simulink model "dynamic_model_soft_robot"  (R2018a)
settings: Solver=ode4  StartTime=0.0  StopTime=t_span  FixedStep=dt  RelTol=1e-3
values from neighbouring files (symbols this model uses):
  alpha0 = 0    [data_simulate_srm_dynamic_model.m]
  c1 = 0.12    [data_simulate_srm_dynamic_model.m]
  c2 = 5.93e-7    (= 5.93e-07)    [data_simulate_srm_dynamic_model.m]
  c3 = 5.93e-7    (= 5.93e-07)    [data_simulate_srm_dynamic_model.m]
  d0 = 0.0644    [data_simulate_srm_dynamic_model.m]
  dq_0 = [0; 0; 500]    [data_simulate_srm_dynamic_model.m]
  dt = 1.00e-03    (= 0.001)    [data_simulate_srm_dynamic_model.m]    (also in simulateSoftRobot.m)
  g = 9.81    [data_simulate_srm_dynamic_model.m]    (also in simulateSoftRobot.m)
  m = 0.0494    [data_simulate_srm_dynamic_model.m]    (also in simulateSoftRobot.m)
  noise_ddq = 0*[1e-4, 1e-4, 1e-4]    [data_simulate_srm_dynamic_model.m]
  noise_dq = 0*[1e-4, 1e-4, 1e-4]    [data_simulate_srm_dynamic_model.m]
  noise_q = 0*[1e-6, 1e-1, 1e-1]    [data_simulate_srm_dynamic_model.m]
  p_true = [b1; b2; b3; b4; b5; b6]    [data_simulate_srm_dynamic_model.m]
  q_0 = [d0; 10; .1]    [data_simulate_srm_dynamic_model.m]
  r = 0.0235    [data_simulate_srm_dynamic_model.m]    (also in simulateSoftRobot.m = 0.02)
libraries: dspinverses x1
(part 1 of 3)
settings Model: Creator=s118759  LastModifiedBy=s118759
settings CodeAppCC: StateflowObjectComments=on

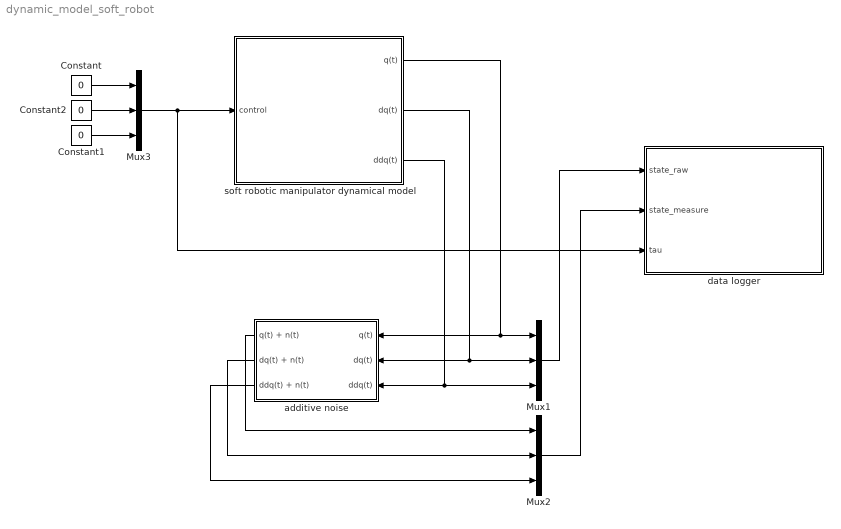
== system dynamic_model_soft_robot ==
  Constant : Constant  Value=0
  Constant1 : Constant  Value=0
  Constant2 : Constant  Value=0
  Mux1 : Mux  Inputs=3
  Mux2 : Mux  Inputs=3
  Mux3 : Mux  Inputs=3
  "additive noise " : Subsystem
  data logger : Subsystem
  soft robotic manipulator dynamical model : Subsystem
  wires:
  soft robotic manipulator dynamical model/1(q(t)) -> "additive noise "/1(q(t)), Mux1/1
  soft robotic manipulator dynamical model/2("dq(t) ") -> Mux1/2, "additive noise "/2(dq(t))
  soft robotic manipulator dynamical model/3("ddq(t) ") -> "additive noise "/3(ddq(t)), Mux1/3
  Mux1/1 -> data logger/1("state_raw ")
  "additive noise "/1(q(t) + n(t)) -> Mux2/1
  "additive noise "/2(dq(t) + n(t)) -> Mux2/2
  "additive noise "/3(ddq(t) + n(t)) -> Mux2/3
  Mux2/1 -> data logger/2(state_measure)
  Mux3/1 -> data logger/3(tau), soft robotic manipulator dynamical model/1("control ")
  Constant/1 -> Mux3/1
  Constant1/1 -> Mux3/3
  Constant2/1 -> Mux3/2

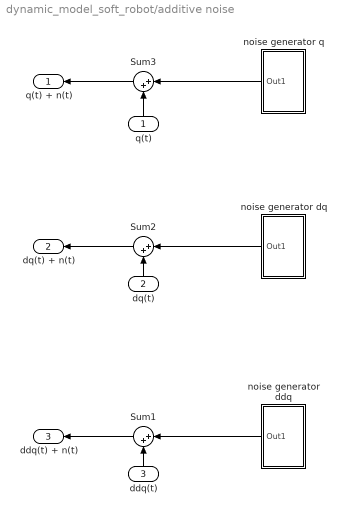
== system dynamic_model_soft_robot/additive noise  ==
  q(t) : Inport
  dq(t) : Inport  Port=2
  ddq(t) : Inport  Port=3
  Sum1 : Sum  Inputs=|++
  Sum2 : Sum  Inputs=|++
  Sum3 : Sum  Inputs=|++
  noise generator ddq : Subsystem
  noise generator dq : Subsystem
  noise generator q : Subsystem
  q(t) + n(t) : Outport
  dq(t) + n(t) : Outport  Port=2
  ddq(t) + n(t) : Outport  Port=3
  wires:
  Sum2/1 -> dq(t) + n(t)/1
  q(t)/1 -> Sum3/2
  Sum3/1 -> q(t) + n(t)/1
  dq(t)/1 -> Sum2/2
  Sum1/1 -> ddq(t) + n(t)/1
  ddq(t)/1 -> Sum1/2
  noise generator q/1(Out1) -> Sum3/1
  noise generator dq/1(Out1) -> Sum2/1
  noise generator ddq/1(Out1) -> Sum1/1

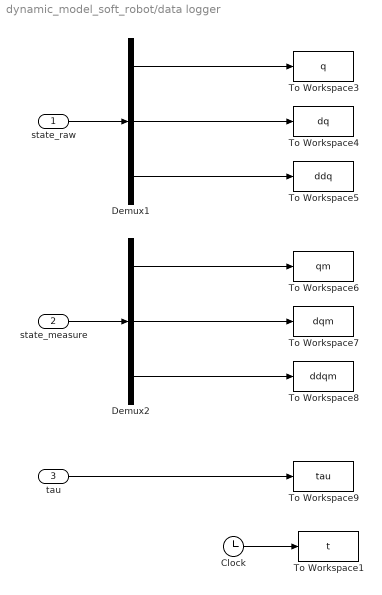
== system dynamic_model_soft_robot/data logger ==
  "state_raw " : Inport
  state_measure : Inport  Port=2
  tau : Inport  Port=3
  Clock : Clock
  Demux1 : Demux  Outputs=3
  Demux2 : Demux  Outputs=3
  To Workspace1 : ToWorkspace  VariableName=t  SampleTime=-1
      settings: Save2DSignal=2-D array (concatenate along first dimension)
  To Workspace3 : ToWorkspace  VariableName=q  SampleTime=-1
      settings: Save2DSignal=2-D array (concatenate along first dimension)
  To Workspace4 : ToWorkspace  VariableName=dq  SampleTime=-1
      settings: Save2DSignal=2-D array (concatenate along first dimension)
  To Workspace5 : ToWorkspace  VariableName=ddq  SampleTime=-1
      settings: Save2DSignal=2-D array (concatenate along first dimension)
  To Workspace6 : ToWorkspace  VariableName=qm  SampleTime=-1
      settings: Save2DSignal=2-D array (concatenate along first dimension)
  To Workspace7 : ToWorkspace  VariableName=dqm  SampleTime=-1
      settings: Save2DSignal=2-D array (concatenate along first dimension)
  To Workspace8 : ToWorkspace  VariableName=ddqm  SampleTime=-1
      settings: Save2DSignal=2-D array (concatenate along first dimension)
  To Workspace9 : ToWorkspace  VariableName=tau  SampleTime=-1
      settings: Save2DSignal=2-D array (concatenate along first dimension)
  wires:
  "state_raw "/1 -> Demux1/1
  Demux1/1 -> To Workspace3/1
  Demux1/2 -> To Workspace4/1
  Demux1/3 -> To Workspace5/1
  state_measure/1 -> Demux2/1
  Demux2/1 -> To Workspace6/1
  Demux2/2 -> To Workspace7/1
  Demux2/3 -> To Workspace8/1
  tau/1 -> To Workspace9/1
  Clock/1 -> To Workspace1/1

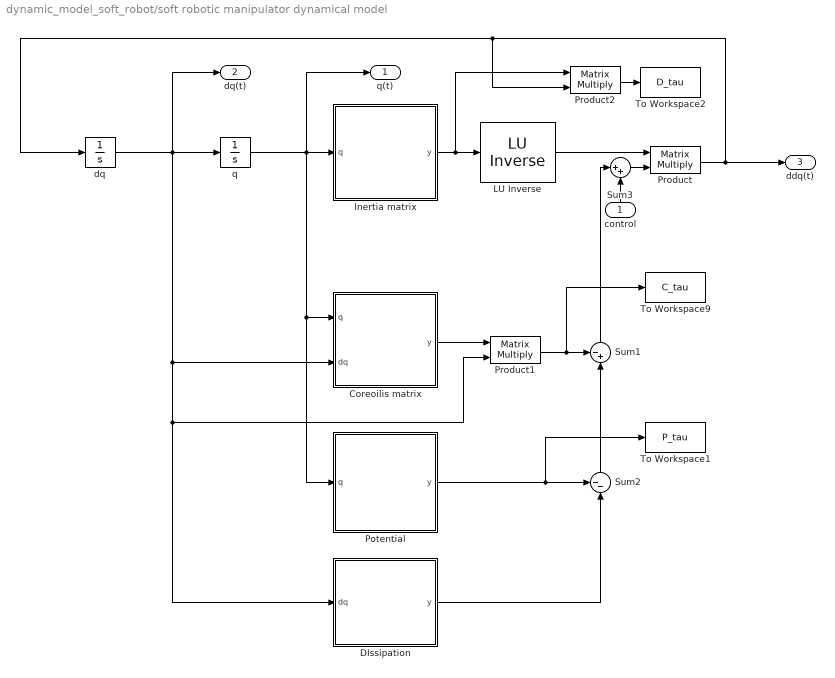
== system dynamic_model_soft_robot/soft robotic manipulator dynamical model ==
  "control " : Inport
  " LU Inverse" : dspinverses/ LU Inverse
      settings: SourceProductName=DSP System Toolbox
  "Coreoilis matrix " : MATLAB Function  TreatAsAtomicUnit=on
  "DIssipation " : MATLAB Function  TreatAsAtomicUnit=on
  "Inertia matrix " : MATLAB Function  TreatAsAtomicUnit=on
  Potential : MATLAB Function  TreatAsAtomicUnit=on
  Product : Product  Multiplication=Matrix(*)
  Product1 : Product  Multiplication=Matrix(*)
  Product2 : Product  Multiplication=Matrix(*)
  Sum1 : Sum  Inputs=-+|
  Sum2 : Sum  Inputs=--|
  Sum3 : Sum  Inputs=|++
  To Workspace1 : ToWorkspace  VariableName=P_tau  SampleTime=-1
      settings: Save2DSignal=2-D array (concatenate along first dimension)
  To Workspace2 : ToWorkspace  VariableName=D_tau  SampleTime=-1
      settings: Save2DSignal=2-D array (concatenate along first dimension)
  To Workspace9 : ToWorkspace  VariableName=C_tau  SampleTime=-1
      settings: Save2DSignal=2-D array (concatenate along first dimension)
  dq : Integrator  InitialCondition=dq_0
  q : Integrator  InitialCondition=q_0
  q(t) : Outport
  "dq(t) " : Outport  Port=2
  "ddq(t) " : Outport  Port=3
  wires:
  "Inertia matrix "/1(y) -> Product2/1, " LU Inverse"/1
  " LU Inverse"/1 -> Product/1
  Potential/1(y) -> To Workspace1/1, Sum2/1
  Sum2/1 -> Sum1/2
  dq/1 -> "dq(t) "/1, q/1, "Coreoilis matrix "/2(dq), "DIssipation "/1(dq), Product1/2
  "control "/1 -> Sum3/2
  "DIssipation "/1(y) -> Sum2/2
  "Coreoilis matrix "/1(y) -> Product1/1
  Sum3/1 -> Product/2
  Product/1 -> "ddq(t) "/1, Product2/2, dq/1
  Sum1/1 -> Sum3/1
  q/1 -> "Inertia matrix "/1(q), q(t)/1, "Coreoilis matrix "/1(q), Potential/1(q)
  Product2/1 -> To Workspace2/1
  Product1/1 -> Sum1/1, To Workspace9/1

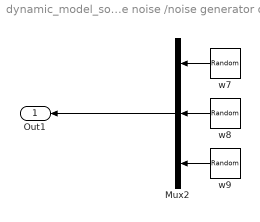
== system dynamic_model_soft_robot/additive noise /noise generator ddq ==
  Mux2 : Mux  Inputs=3
  w7 : RandomNumber  Variance=noise_ddq(1)  SampleTime=dt
  w8 : RandomNumber  Variance=noise_ddq(2)  SampleTime=dt
  w9 : RandomNumber  Variance=noise_ddq(3)  SampleTime=dt
  Out1 : Outport
  wires:
  w7/1 -> Mux2/1
  w9/1 -> Mux2/3
  w8/1 -> Mux2/2
  Mux2/1 -> Out1/1

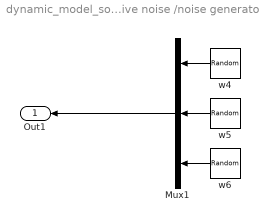
== system dynamic_model_soft_robot/additive noise /noise generator dq ==
  Mux1 : Mux  Inputs=3
  w4 : RandomNumber  Variance=noise_dq(1)  SampleTime=dt
  w5 : RandomNumber  Variance=noise_dq(2)  SampleTime=dt
  w6 : RandomNumber  Variance=noise_dq(3)  SampleTime=dt
  Out1 : Outport
  wires:
  w6/1 -> Mux1/3
  w5/1 -> Mux1/2
  w4/1 -> Mux1/1
  Mux1/1 -> Out1/1

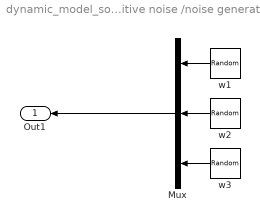
== system dynamic_model_soft_robot/additive noise /noise generator q ==
  Mux : Mux  Inputs=3
  w1 : RandomNumber  Variance=noise_q(1)  SampleTime=dt
  w2 : RandomNumber  Variance=noise_q(2)  SampleTime=dt
  w3 : RandomNumber  Variance=noise_q(3)  SampleTime=dt
  Out1 : Outport
  wires:
  w3/1 -> Mux/3
  w2/1 -> Mux/2
  w1/1 -> Mux/1
  Mux/1 -> Out1/1
